simulink model "chap6_4sim"  (Simulink 8.1)
settings: Solver=ode45  StartTime=0.0  StopTime=10  RelTol=1e-3
settings Model: Creator=Administrator  LastModifiedBy=liujk
settings DataIOCC: SignalLoggingName=sigsOut
settings OptimizationCC: InitFltsAndDblsToZero=on
settings DebuggingCC: SaveWithParameterizedLinksMsg=none  SignalResolutionControl=TryResolveAllWithWarning  SolverPrmCheckMsg=none  MultiTaskDSMMsg=warning  MultiTaskCondExecSysMsg=none  StrictBusMsg=None
settings HardwareCC: TargetUnknown=on
settings RTWCC: IncludeERTFirstTime=on
settings GRTTargetCC: TargetFcnLib=ansi_tfl_tmw.mat

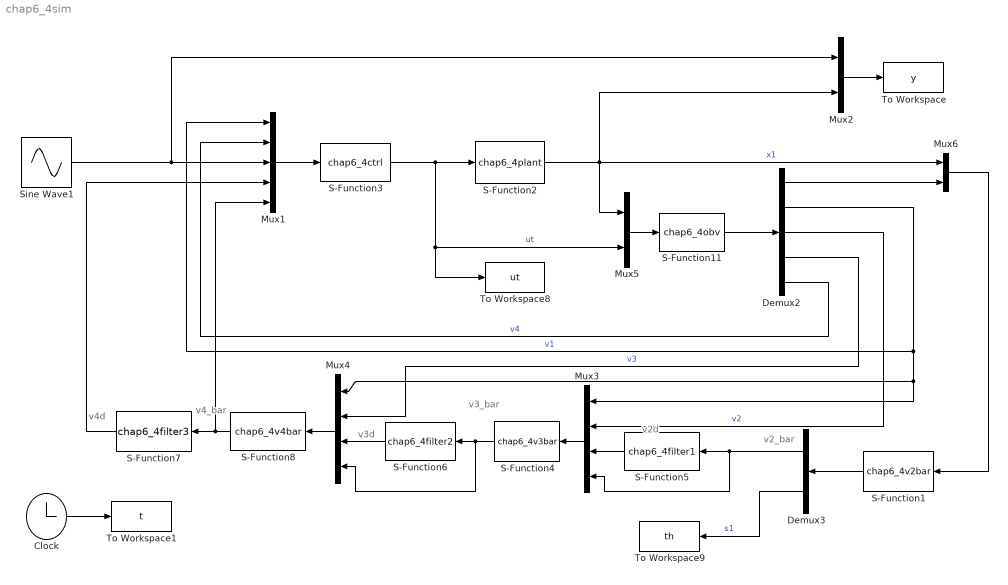
== system chap6_4sim ==
  note: v2d
  note: v2_bar
  note: v3_bar
  note: v3d
  note: v4_bar
  note: v4d
  Clock : Clock
  Demux2 : Demux  Outputs=5
  Demux3 : Demux  Outputs=2
  Mux1 : Mux  Inputs=5
  Mux2 : Mux  Inputs=2
  Mux3 : Mux
  Mux4 : Mux
  Mux5 : Mux  Inputs=2
  Mux6 : Mux  Inputs=2
  S-Function1 : S-Function  FunctionName=chap6_4v2bar  EnableBusSupport=off
  S-Function11 : S-Function  FunctionName=chap6_4obv  EnableBusSupport=off
  S-Function2 : S-Function  FunctionName=chap6_4plant  EnableBusSupport=off
  S-Function3 : S-Function  FunctionName=chap6_4ctrl  EnableBusSupport=off
  S-Function4 : S-Function  FunctionName=chap6_4v3bar  EnableBusSupport=off
  S-Function5 : S-Function  FunctionName=chap6_4filter1  EnableBusSupport=off
  S-Function6 : S-Function  FunctionName=chap6_4filter2  EnableBusSupport=off
  S-Function7 : S-Function  FunctionName=chap6_4filter3  EnableBusSupport=off
  S-Function8 : S-Function  FunctionName=chap6_4v4bar  EnableBusSupport=off
  Sine Wave1 : Sin  SampleTime=0
  To Workspace : ToWorkspace  VariableName=y  SampleTime=-1
  To Workspace1 : ToWorkspace  VariableName=t  SampleTime=-1
  To Workspace8 : ToWorkspace  VariableName=ut  SampleTime=-1
  To Workspace9 : ToWorkspace  VariableName=th  SampleTime=-1
  wires:
  Clock/1 -> To Workspace1/1
  Mux1/1 -> S-Function3/1
  Sine Wave1/1 -> Mux2/1, Mux1/3
  S-Function2/1 -> Mux5/1, Mux6/1, Mux2/2  "x1"
  Mux2/1 -> To Workspace/1
  Mux3/1 -> S-Function4/1
  S-Function8/1 -> S-Function7/1, Mux1/5
  Mux4/1 -> S-Function8/1
  S-Function6/1 -> Mux4/3
  S-Function7/1 -> Mux1/4
  S-Function3/1 -> S-Function2/1, Mux5/2, To Workspace8/1  "ut"
  Mux5/1 -> S-Function11/1
  S-Function11/1 -> Demux2/1
  Mux6/1 -> S-Function1/1
  S-Function1/1 -> Demux3/1
  Demux3/1 -> S-Function5/1, Mux3/4
  S-Function5/1 -> Mux3/3
  S-Function4/1 -> S-Function6/1, Mux4/4
  Demux3/2 -> To Workspace9/1  "s1"
  Demux2/1 -> Mux6/2
  Demux2/2 -> Mux3/1, Mux4/1, Mux1/1  "v1"
  Demux2/3 -> Mux3/2  "v2"
  Demux2/4 -> Mux4/2  "v3"
  Demux2/5 -> Mux1/2  "v4"
